simulink model "fva_ut"  (Simulink 8.1)
settings: Solver=FixedStepDiscrete  StartTime=0.0  StopTime=Inf  FixedStep=0.005  RelTol=1e-3
undefined symbols (not defined in the file or in its folder): C_TICK_TIME_S
libraries: fva x1, hcu_lib x1
settings Model: Creator=xsellart  LastModifiedBy=AT015555
settings DataIOCC: SignalLoggingSaveFormat=Dataset
settings OptimizationCC: ExpressionDepthLimit=128
settings DebuggingCC: FcnCallInpInsideContextMsg=EnableAllAsError
settings GRTTargetCC: CombineOutputUpdateFcns=on  GRTInterface=off

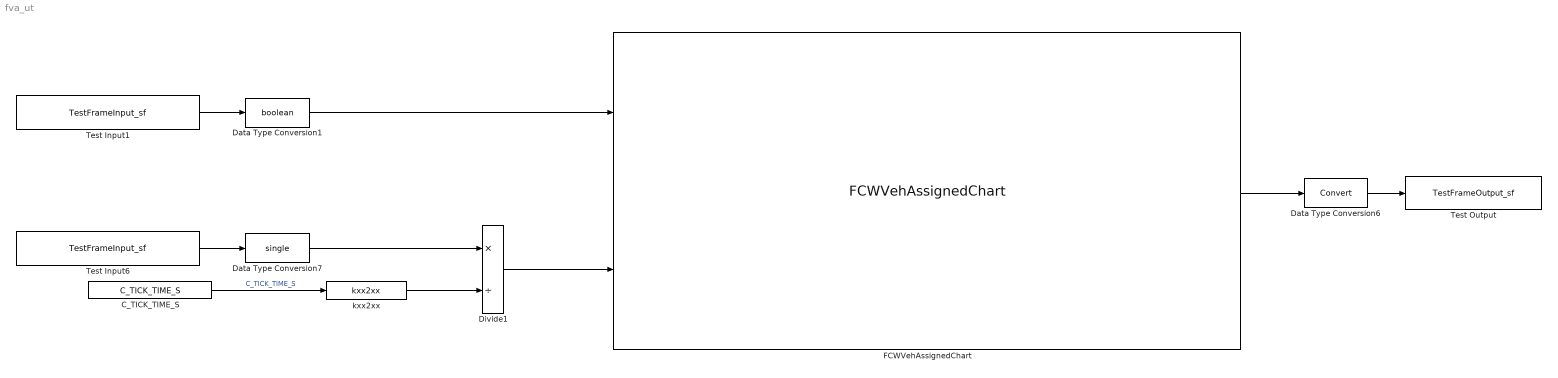
== system fva_ut ==
  C_TICK_TIME_S : Constant  Value=C_TICK_TIME_S
  Data Type Conversion1 : DataTypeConversion  OutDataTypeStr=boolean
  Data Type Conversion6 : DataTypeConversion
  Data Type Conversion7 : DataTypeConversion  OutDataTypeStr=single
  Divide1 : Product  Inputs=*/
  FCWVehAssignedChart : fva/FCWVehAssignedChart
  Test Input1 : S-Function  FunctionName=TestFrameInput_sf  Parameters=varname,sampletime  EnableBusSupport=off  mask(Test Input){varname=VIFO_FCWTargetVehAssigned_flg, sampletime=0.005}
      mask prompts: varname "Name:"; sampletime "Sample Time:"
      mask help: Outputs the value of a Test Input variable from an Excel spreadsheet when used with the runsiltest script. Otherwise outputs 0.
      mask Display: fprintf('Test Input:\n%s',varname);
  Test Input6 : S-Function  FunctionName=TestFrameInput_sf  Parameters=varname,sampletime  EnableBusSupport=off  mask(Test Input){varname=KJUD_FCWVehAssignTimer_ms, sampletime=0.005}
      mask prompts: varname "Name:"; sampletime "Sample Time:"
      mask help: Outputs the value of a Test Input variable from an Excel spreadsheet when used with the runsiltest script. Otherwise outputs 0.
      mask Display: fprintf('Test Input:\n%s',varname);
  Test Output : S-Function  FunctionName=TestFrameOutput_sf  Parameters=varname,sampletime  EnableBusSupport=off  mask(Test Output){varname=VJUD_FCWVehAssigned_flg, sampletime=-1}
      mask prompts: varname "Name:"; sampletime "Sample Time:"
      mask help: Samples the value of a Test Output variable from an Excel spreadsheet when used with the runsiltest script. Otherwise does nothing.
      mask Display: fprintf('Test Output:\n%s',varname);
  kxx2xx : hcu_lib/kxx2xx
  wires:
  Test Input1/1 -> Data Type Conversion1/1
  Data Type Conversion1/1 -> FCWVehAssignedChart/1
  FCWVehAssignedChart/1 -> Data Type Conversion6/1
  Data Type Conversion6/1 -> Test Output/1
  Test Input6/1 -> Data Type Conversion7/1
  Data Type Conversion7/1 -> Divide1/1
  kxx2xx/1 -> Divide1/2
  C_TICK_TIME_S/1 -> kxx2xx/1  "C_TICK_TIME_S"
  Divide1/1 -> FCWVehAssignedChart/2
